simulink model "tailSim"  (R2020b)
settings: Solver=ode45  StartTime=0.0  StopTime=simTime  FixedStep=0.0005  RelTol=1e-6  AbsTol=1e-9
values from neighbouring files (symbols this model uses):
  p1_end__1 = [-l_t/2; 0; 0]    [cheetahAnim.m]    (also in cheetahEOM.m; tailAnim.m = [-L/2; 0; 0]; tailEOM.m = [-L/2; 0; 0])
  pF = [pF1_1__1, pF1_2__1, pF2_1__2, pF2_2__2]    [tailAnim.m]
  tau_max = 30    [cheetahTrajOpt.m]    (also in tailTrajOpt.m)
libraries: simulink x15
settings Model: Creator=ricky  LastModifiedBy=ricky
settings SFSimCC: CustomCodeUndefinedFunction=UseInterfaceOnly

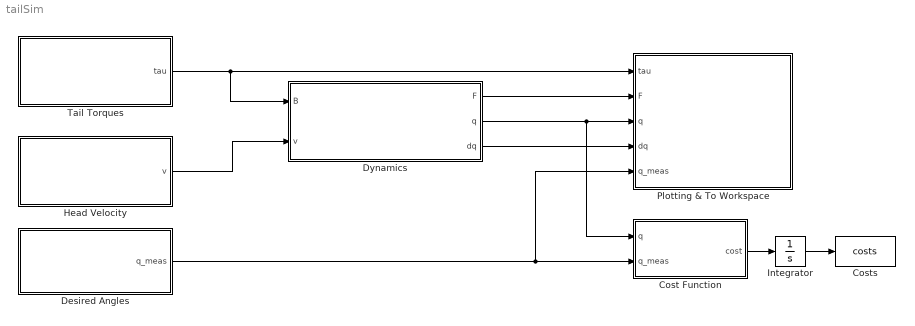
== system tailSim ==
  Cost Function : MATLAB Function  TreatAsAtomicUnit=on
  Costs : ToWorkspace  VariableName=costs  SampleTime=0.001
  Desired Angles : Subsystem
  Dynamics : Subsystem
  Head Velocity : Subsystem
  Integrator : Integrator
  Plotting & To Workspace : Subsystem
  Tail Torques : Subsystem
  wires:
  Dynamics/2(q) -> Cost Function/1(q), Plotting & To Workspace/3(q)
  Cost Function/1(cost) -> Integrator/1
  Integrator/1 -> Costs/1
  Dynamics/1(F) -> Plotting & To Workspace/2(F)
  Dynamics/3(dq) -> Plotting & To Workspace/4(dq)
  Tail Torques/1(tau) -> Dynamics/1(B), Plotting & To Workspace/1(tau)
  Desired Angles/1(q_meas) -> Plotting & To Workspace/5(q_meas), Cost Function/2(q_meas)
  Head Velocity/1(v) -> Dynamics/2(v)

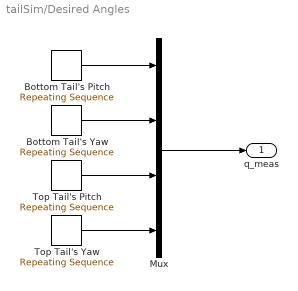
== system tailSim/Desired Angles ==
  Bottom Tail's Pitch : simulink/Sources/Repeating Sequence  rep_seq_t=time  rep_seq_y=th1_meas
  Bottom Tail's Yaw : simulink/Sources/Repeating Sequence  rep_seq_t=time  rep_seq_y=psi1_meas
  Mux : Mux
  Top Tail's Pitch : simulink/Sources/Repeating Sequence  rep_seq_t=time  rep_seq_y=th2_meas
  Top Tail's Yaw : simulink/Sources/Repeating Sequence  rep_seq_t=time  rep_seq_y=psi2_meas
  q_meas : Outport
  wires:
  Bottom Tail's Pitch/1 -> Mux/1
  Bottom Tail's Yaw/1 -> Mux/2
  Top Tail's Yaw/1 -> Mux/4
  Top Tail's Pitch/1 -> Mux/3
  Mux/1 -> q_meas/1

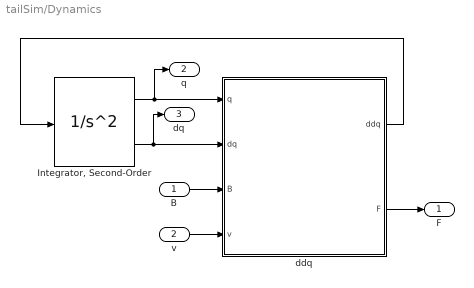
== system tailSim/Dynamics ==
  B : Inport
  v : Inport  Port=2
  "Integrator, Second-Order" : SecondOrderIntegrator  ICX=q0  ICDXDT=dq0
  ddq : MATLAB Function  TreatAsAtomicUnit=on
  F : Outport
  q : Outport  Port=2
  dq : Outport  Port=3
  wires:
  "Integrator, Second-Order"/2 -> dq/1, ddq/2(dq)
  "Integrator, Second-Order"/1 -> q/1, ddq/1(q)
  B/1 -> ddq/3(B)
  ddq/2(F) -> F/1
  ddq/1(ddq) -> "Integrator, Second-Order"/1
  v/1 -> ddq/4(v)

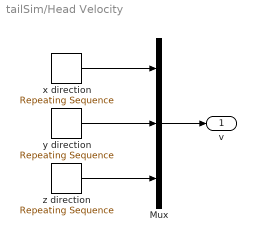
== system tailSim/Head Velocity ==
  Mux : Mux  Inputs=3
  x direction : simulink/Sources/Repeating Sequence  rep_seq_t=time  rep_seq_y=vx
  y direction : simulink/Sources/Repeating Sequence  rep_seq_t=time  rep_seq_y=vy
  z direction : simulink/Sources/Repeating Sequence  rep_seq_t=time  rep_seq_y=vz
  v : Outport
  wires:
  x direction/1 -> Mux/1
  y direction/1 -> Mux/2
  z direction/1 -> Mux/3
  Mux/1 -> v/1

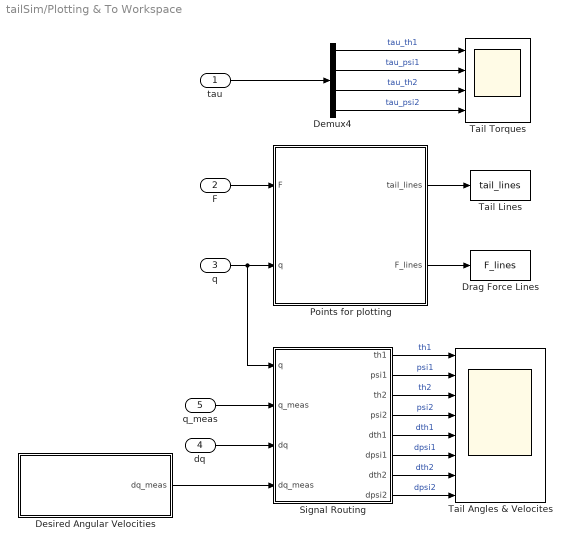
== system tailSim/Plotting & To Workspace ==
  tau : Inport
  F : Inport  Port=2
  q : Inport  Port=3
  dq : Inport  Port=4
  q_meas : Inport  Port=5
  Demux4 : Demux
  Desired Angular Velocities : Subsystem
  Drag Force Lines : ToWorkspace  VariableName=F_lines  SampleTime=-1
  Points for plotting : MATLAB Function  TreatAsAtomicUnit=on
  Signal Routing : MATLAB Function  TreatAsAtomicUnit=on
  Tail Angles & Velocites : Scope  NumInputPorts=8
  "Tail Lines " : ToWorkspace  VariableName=tail_lines  SampleTime=-1
  Tail Torques : Scope  NumInputPorts=4
  wires:
  F/1 -> Points for plotting/1(F)
  Points for plotting/1(tail_lines) -> "Tail Lines "/1
  q/1 -> Signal Routing/1(q), Points for plotting/2(q)
  Points for plotting/2(F_lines) -> Drag Force Lines/1
  dq/1 -> Signal Routing/3(dq)
  q_meas/1 -> Signal Routing/2(q_meas)
  Signal Routing/5(dth1) -> Tail Angles & Velocites/5  "dth1"
  Signal Routing/6(dpsi1) -> Tail Angles & Velocites/6  "dpsi1"
  Signal Routing/8(dpsi2) -> Tail Angles & Velocites/8  "dpsi2"
  Signal Routing/4(psi2) -> Tail Angles & Velocites/4  "psi2"
  Signal Routing/3(th2) -> Tail Angles & Velocites/3  "th2"
  Signal Routing/2(psi1) -> Tail Angles & Velocites/2  "psi1"
  Signal Routing/1(th1) -> Tail Angles & Velocites/1  "th1"
  Signal Routing/7(dth2) -> Tail Angles & Velocites/7  "dth2"
  Desired Angular Velocities/1(dq_meas) -> Signal Routing/4(dq_meas)
  Demux4/3 -> Tail Torques/3  "tau_th2"
  Demux4/4 -> Tail Torques/4  "tau_psi2"
  Demux4/2 -> Tail Torques/2  "tau_psi1"
  Demux4/1 -> Tail Torques/1  "tau_th1"
  tau/1 -> Demux4/1

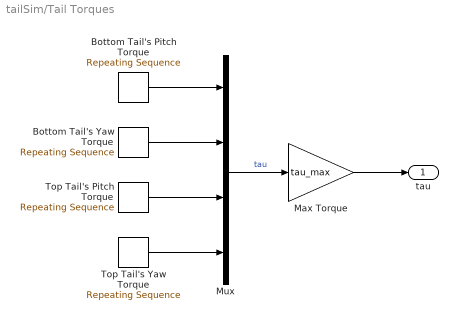
== system tailSim/Tail Torques ==
  Bottom Tail's Pitch Torque : simulink/Sources/Repeating Sequence  rep_seq_t=time_tau  rep_seq_y=tau1_th
  Bottom Tail's Yaw Torque : simulink/Sources/Repeating Sequence  rep_seq_t=time_tau  rep_seq_y=tau1_psi
  Max Torque : Gain  Gain=tau_max
  Mux : Mux
  Top Tail's Pitch Torque : simulink/Sources/Repeating Sequence  rep_seq_t=time_tau  rep_seq_y=tau2_th
  Top Tail's Yaw Torque : simulink/Sources/Repeating Sequence  rep_seq_t=time_tau  rep_seq_y=tau2_psi
  tau : Outport
  wires:
  Bottom Tail's Pitch Torque/1 -> Mux/1
  Bottom Tail's Yaw Torque/1 -> Mux/2
  Top Tail's Pitch Torque/1 -> Mux/3
  Top Tail's Yaw Torque/1 -> Mux/4
  Mux/1 -> Max Torque/1  "tau"
  Max Torque/1 -> tau/1

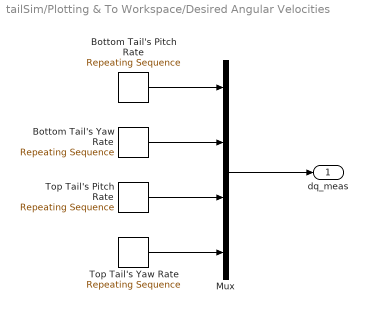
== system tailSim/Plotting & To Workspace/Desired Angular Velocities ==
  Bottom Tail's Pitch Rate : simulink/Sources/Repeating Sequence  rep_seq_t=time  rep_seq_y=dth1_meas
  Bottom Tail's Yaw Rate : simulink/Sources/Repeating Sequence  rep_seq_t=time  rep_seq_y=dpsi1_meas
  Mux : Mux
  Top Tail's Pitch Rate : simulink/Sources/Repeating Sequence  rep_seq_t=time  rep_seq_y=dth2_meas
  Top Tail's Yaw Rate : simulink/Sources/Repeating Sequence  rep_seq_t=time  rep_seq_y=dpsi2_meas
  dq_meas : Outport
  wires:
  Bottom Tail's Pitch Rate/1 -> Mux/1
  Bottom Tail's Yaw Rate/1 -> Mux/2
  Top Tail's Yaw Rate/1 -> Mux/4
  Top Tail's Pitch Rate/1 -> Mux/3
  Mux/1 -> dq_meas/1

== matlab function tailSim/Cost Function ==
  data: q input; cost output; q_meas input
function cost = cost(q, q_meas)
    
    e_q  = q_meas - q;
    cost = e_q'*e_q;
end

== matlab function tailSim/Plotting & To Workspace/Points for plotting ==
  data: F input; q input; tail_lines output; pF parameter; F_lines output; p1_end__1 parameter
function [tail_lines, F_lines] = points4plot(F, q, pF, p1_end__1)
    
    R_0__1 = RotZ(q(2)) * RotY(q(1));
    R_1__0 = R_0__1'; % Rotation of bottom tail into body
    R_2__0 = (RotZ(q(4)) * RotY(q(3)) * R_0__1)';

    % tail point locations
    p1_end__0 = R_1__0 * p1_end__1;
    p2_end__0 = p1_end__0 + R_2__0 * p1_end__1;

    tail1 = [zeros(3, 1), p1_end__0];
    tail2 = [p1_end__0, p2_end__0];
    tail_lines = reshape([tail1, tail2], [3, 2, 2]);
    
    % drag force locations
    pF1_1__0 = R_1__0 * pF(:, 1);
    pF1_2__0 = R_1__0 * pF(:, 2);
    pF2_1__0 = p1_end__0 + R_2__0 * pF(:, 3);
    pF2_2__0 = p1_end__0 + R_2__0 * pF(:, 4);
    
    F = F/25;
    f1 = [pF1_1__0, F(:, 1)];
    f2 = [pF1_2__0, F(:, 2)];
    f3 = [pF2_1__0, F(:, 3)];
    f4 = [pF2_2__0, F(:, 4)];
    F_lines = reshape([f1, f2, f3, f4], [3, 2, 4]);
end
function rot = RotX(th)
    rot = [[1     0       0   ]
           [0  cos(th) sin(th)]
           [0 -sin(th) cos(th)]];
end
% function rot = RotY(th) % standard rotation about y
%     rot = [[ cos(th) 0 sin(th)]
%            [    0    1    0   ]
%            [-sin(th) 0 cos(th)]];
% end
function rot = RotY(th) % Liam's rotation about y
    rot = [[ cos(th) 0 -sin(th)]
           [    0    1    0   ]
           [sin(th) 0 cos(th)]];
end
function rot = RotZ(th)
    rot = [[ cos(th) sin(th) 0]
           [-sin(th) cos(th) 0]
           [    0       0    1]];
end

== matlab function tailSim/Plotting & To Workspace/Signal Routing ==
  data: q input; th1 output; q_meas input; dq input; dq_meas input; psi1 output; th2 output; psi2 output; dth1 output; dpsi1 output; dth2 output; dpsi2 output
function [th1, psi1, th2, psi2, dth1, dpsi1, dth2, dpsi2] = route(q, q_meas, dq, dq_meas)
    th1  = [q(1), q_meas(1)];
    psi1 = [q(2), q_meas(2)];
    th2  = [q(3), q_meas(3)];
    psi2 = [q(4), q_meas(4)];
    
    dth1  = [dq(1), dq_meas(1)];
    dpsi1 = [dq(2), dq_meas(2)];
    dth2  = [dq(3), dq_meas(3)];
    dpsi2 = [dq(4), dq_meas(4)];
end

== matlab function tailSim/Dynamics/ddq ==
  data: ddq output; F output; q input; dq input; B input; Cd parameter; v input
function [ddq, F]  = ddq(q, dq, B, Cd, v)
    coder.extrinsic('tailMCGQ');
    coder.extrinsic('tailDragForces');
    
    F1_1 = zeros(3, 1);
    F1_2 = F1_1;
    F2_1 = F1_1;
    F2_2 = F1_1;
    [F1_1, F1_2, F2_1, F2_2] = tailDragForces(q, dq, Cd, v);
    F = [F1_1, F1_2, F2_1, F2_2];
    
    M = zeros(4, 4);
    C = zeros(4, 1);
    G = C;
    Q = C;
    [M, C, G, Q] = tailMCGQ(q, dq, F);
    
    ddq = M\(B + Q - G - C);
end
